simulink model "gesamtmodell"  (Simulink 7.9)
settings: Solver=ode45  StartTime=0.0  StopTime=6.5  RelTol=1e-3
values from neighbouring files (symbols this model uses):
  bias = [0;0;0]    [init.m]
  g = 9.81    [init.m]
  Kd = 4    [init.m]
  Ki = 0.01    [init.m]
  Kp = 5    [init.m]
  l_1 = 18    [init.m]
  l_2 = 46.18    [init.m]
  l_3 = 3.75    [init.m]
  m = 1.863    [init.m]
  omega_0 = 1.5    [init.m]
  xi = 1    [init.m]
libraries: simulink x4
settings Model: Creator=Matthias  LastModifiedBy=Matthias

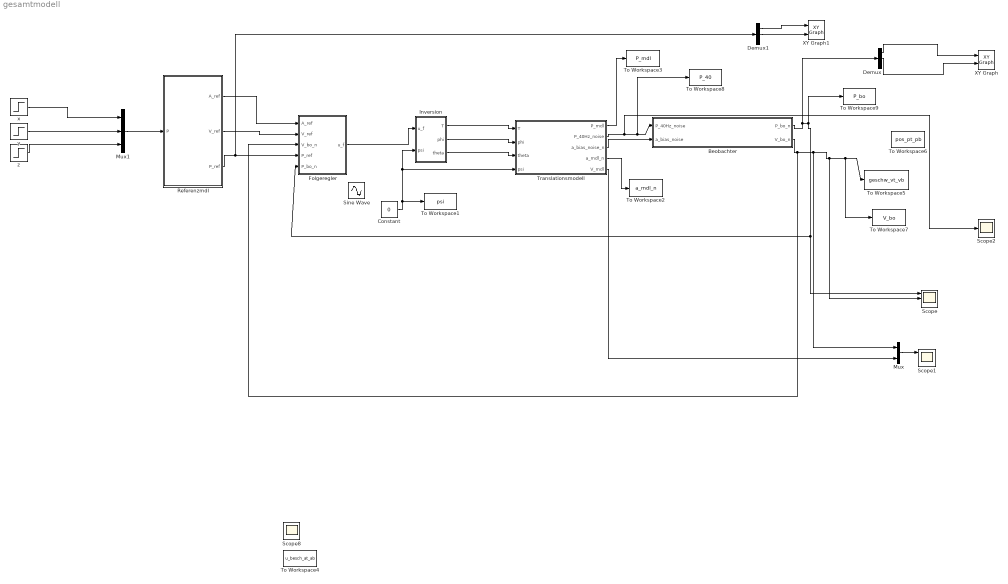
== system gesamtmodell ==
  Beobachter : Subsystem
  Constant : Constant  Value=0
  Demux : Demux  Outputs=3
  Demux1 : Demux  Outputs=3
  Folgeregler : Subsystem
  Inversion : Subsystem
  Mux : Mux  Inputs=2
  Mux1 : Mux  Inputs=3
  Referenzmdl : Subsystem
  Scope : Scope  NumInputPorts=3
      settings: TimeRange=7  YMin=-5~-5~-5  YMax=5~5~5
  Scope1 : Scope  NumInputPorts=3
      settings: YMin=-1.25~-5~-5  YMax=0.75~5~5
  Scope2 : Scope
      settings: SaveName=ScopeData6
  Scope8 : Scope
      settings: SaveName=ScopeData11
  Sine Wave : Sin  SampleTime=0
  To Workspace1 : ToWorkspace  VariableName=psi  SampleTime=-1  SaveFormat=Structure With Time
  To Workspace2 : ToWorkspace  VariableName=a_mdl_n  SampleTime=-1  SaveFormat=Structure With Time
  To Workspace3 : ToWorkspace  VariableName=P_mdl  SampleTime=-1  SaveFormat=Structure With Time
  To Workspace4 : ToWorkspace  VariableName=u_besch_at_ab  SampleTime=-1  SaveFormat=Structure With Time
  To Workspace5 : ToWorkspace  VariableName=geschw_vt_vb  SampleTime=-1  SaveFormat=Structure With Time
  To Workspace6 : ToWorkspace  VariableName=pos_pt_pb  SampleTime=-1  SaveFormat=Structure With Time
  To Workspace7 : ToWorkspace  VariableName=V_bo  SampleTime=-1  SaveFormat=Structure With Time
  To Workspace8 : ToWorkspace  VariableName=P_40  SampleTime=-1  SaveFormat=Structure With Time
  To Workspace9 : ToWorkspace  VariableName=P_bo  SampleTime=-1  SaveFormat=Structure With Time
  Translationsmodell : Subsystem
  XY Graph : simulink/Sinks/XY Graph  xmin=-2.5  xmax=0.5  ymin=-0.5  ymax=2.5  st=-1
  XY Graph1 : simulink/Sinks/XY Graph  xmin=-2.5  xmax=0.5  ymin=-0.5  ymax=2.5  st=-1
  x : Step  Time=0.5  After=-2  SampleTime=0
  y : Step  Time=0.5  SampleTime=0
  z : Step  After=0  SampleTime=0
  wires:
  Inversion/1(T) -> Translationsmodell/1(T)
  Inversion/2(phi) -> Translationsmodell/2(phi)
  Inversion/3(theta) -> Translationsmodell/3(theta)
  Translationsmodell/4(a_mdl_n) -> To Workspace2/1
  Translationsmodell/2(P_40Hz_noise) -> Scope2/1, Beobachter/1(P_40Hz_noise), To Workspace8/1
  Translationsmodell/3(a_bias_noise_n) -> Beobachter/2(a_bias_noise)
  Beobachter/2(V_bo_n) -> Scope/2, To Workspace5/1, To Workspace7/1, Mux/1, Folgeregler/3(V_bo_n)
  Mux1/1 -> Referenzmdl/1(P)
  Folgeregler/1(u_f) -> Inversion/1(u_f)
  Referenzmdl/1(A_ref) -> Folgeregler/1(A_ref)
  Referenzmdl/2(V_ref) -> Folgeregler/2(V_ref)
  Referenzmdl/3(P_ref) -> Folgeregler/4(P_ref), Demux1/1
  x/1 -> Mux1/1
  y/1 -> Mux1/2
  z/1 -> Mux1/3
  Translationsmodell/1(P_mdl) -> To Workspace3/1
  Translationsmodell/5(V_mdl) -> Mux/2
  Mux/1 -> Scope1/1
  Beobachter/1(P_bo_n) -> Demux/1, Scope/1, Folgeregler/5(P_bo_n), To Workspace9/1
  Demux/2 -> XY Graph/2
  Demux/1 -> XY Graph/1
  Demux1/1 -> XY Graph1/1
  Demux1/2 -> XY Graph1/2
  Constant/1 -> Inversion/2(psi), Translationsmodell/4(psi), To Workspace1/1

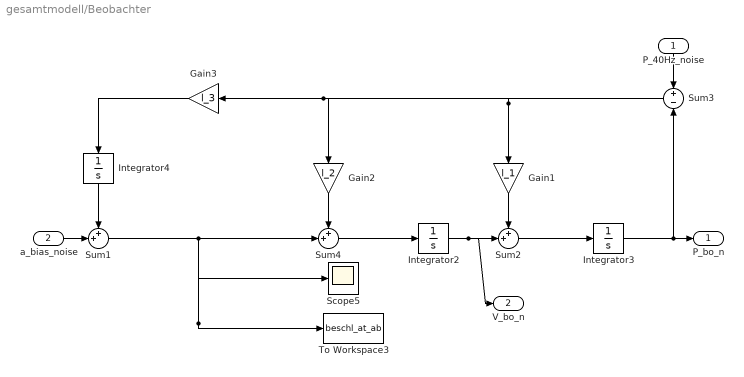
== system gesamtmodell/Beobachter ==
  P_40Hz_noise : Inport
  a_bias_noise : Inport  Port=2
  Gain1 : Gain  Gain=l_1
  Gain2 : Gain  Gain=l_2
  Gain3 : Gain  Gain=l_3
  Integrator2 : Integrator
  Integrator3 : Integrator
  Integrator4 : Integrator
  Scope5 : Scope
      settings: SaveName=ScopeData8
  Sum1 : Sum  Inputs=++|
  Sum2 : Sum  Inputs=++|
  Sum3 : Sum  Inputs=+|-
  Sum4 : Sum  Inputs=++|
  To Workspace3 : ToWorkspace  VariableName=beschl_at_ab  SampleTime=-1  SaveFormat=Structure With Time
  P_bo_n : Outport
  V_bo_n : Outport  Port=2
  wires:
  Gain3/1 -> Integrator4/1
  Sum1/1 -> Sum4/2, Scope5/1, To Workspace3/1
  Integrator4/1 -> Sum1/1
  Gain2/1 -> Sum4/1
  Sum4/1 -> Integrator2/1
  Sum3/1 -> Gain1/1, Gain3/1, Gain2/1
  Gain1/1 -> Sum2/1
  Integrator3/1 -> Sum3/2, P_bo_n/1
  Sum2/1 -> Integrator3/1
  Integrator2/1 -> Sum2/2, V_bo_n/1
  P_40Hz_noise/1 -> Sum3/1
  a_bias_noise/1 -> Sum1/2

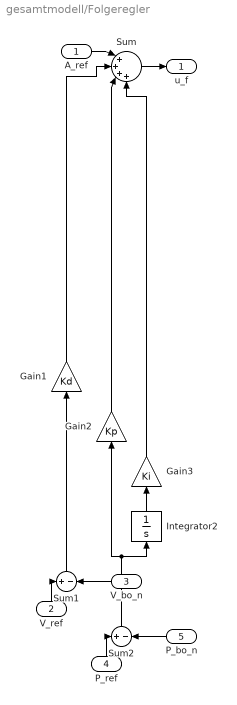
== system gesamtmodell/Folgeregler ==
  A_ref : Inport
  V_ref : Inport  Port=2
  V_bo_n : Inport  Port=3
  P_ref : Inport  Port=4
  P_bo_n : Inport  Port=5
  Gain1 : Gain  Gain=Kd
  Gain2 : Gain  Gain=Kp
  Gain3 : Gain  Gain=Ki
  Integrator2 : Integrator
  Sum : Sum  Inputs=|++++
  Sum1 : Sum  Inputs=+|-
  Sum2 : Sum  Inputs=+|-
  u_f : Outport
  wires:
  Sum1/1 -> Gain1/1
  Sum2/1 -> Gain2/1, Integrator2/1
  Integrator2/1 -> Gain3/1
  V_bo_n/1 -> Sum1/2
  P_bo_n/1 -> Sum2/2
  A_ref/1 -> Sum/1
  Sum/1 -> u_f/1
  V_ref/1 -> Sum1/1
  P_ref/1 -> Sum2/1
  Gain1/1 -> Sum/2
  Gain2/1 -> Sum/3
  Gain3/1 -> Sum/4

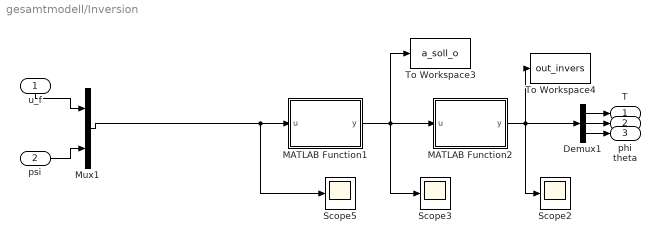
== system gesamtmodell/Inversion ==
  u_f : Inport
  psi : Inport  Port=2
  Demux1 : Demux  Outputs=3
  MATLAB Function1 : MATLAB Function  TreatAsAtomicUnit=on
  MATLAB Function2 : MATLAB Function  TreatAsAtomicUnit=on
  Mux1 : Mux  Inputs=2
  Scope2 : Scope
      settings: SaveName=ScopeData2
  Scope3 : Scope
      settings: SaveName=ScopeData3
  Scope5 : Scope
      settings: SaveName=ScopeData5
  To Workspace3 : ToWorkspace  VariableName=a_soll_o  SampleTime=-1  SaveFormat=Structure With Time
  To Workspace4 : ToWorkspace  VariableName=out_invers  SampleTime=-1  SaveFormat=Structure With Time
  T : Outport
  phi : Outport  Port=2
  theta : Outport  Port=3
  wires:
  Mux1/1 -> MATLAB Function1/1(u), Scope5/1
  MATLAB Function1/1(y) -> MATLAB Function2/1(u), Scope3/1, To Workspace3/1
  MATLAB Function2/1(y) -> Demux1/1, Scope2/1, To Workspace4/1
  u_f/1 -> Mux1/1
  psi/1 -> Mux1/2
  Demux1/1 -> T/1
  Demux1/2 -> phi/1
  Demux1/3 -> theta/1

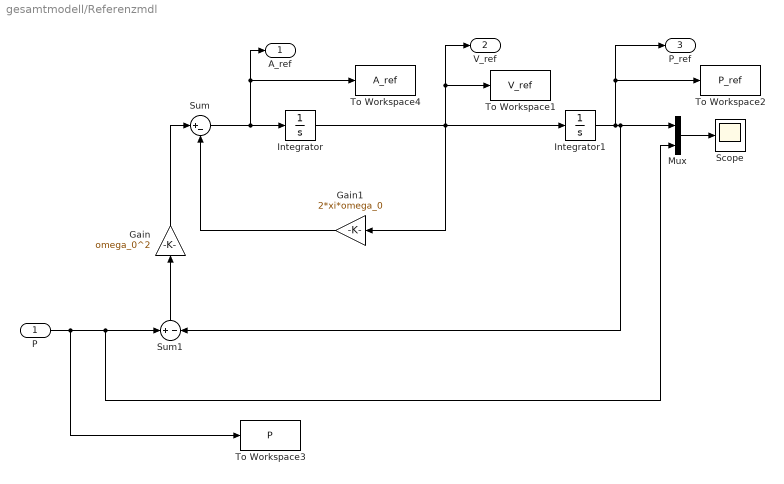
== system gesamtmodell/Referenzmdl ==
  P : Inport
  Gain : Gain  Gain=omega_0^2
  Gain1 : Gain  Gain=2*xi*omega_0
  Integrator : Integrator
  Integrator1 : Integrator
  Mux : Mux  Inputs=2
  Scope : Scope
  Sum : Sum  Inputs=|+-
  Sum1 : Sum  Inputs=+|-
  To Workspace1 : ToWorkspace  VariableName=V_ref  SampleTime=-1  SaveFormat=Structure With Time
  To Workspace2 : ToWorkspace  VariableName=P_ref  SampleTime=-1  SaveFormat=Structure With Time
  To Workspace3 : ToWorkspace  VariableName=P  SampleTime=-1  SaveFormat=Structure With Time
  To Workspace4 : ToWorkspace  VariableName=A_ref  SampleTime=-1  SaveFormat=Structure With Time
  A_ref : Outport
  V_ref : Outport  Port=2
  P_ref : Outport  Port=3
  wires:
  Sum1/1 -> Gain/1
  Gain/1 -> Sum/1
  Sum/1 -> Integrator/1, A_ref/1, To Workspace4/1
  Integrator/1 -> Integrator1/1, Gain1/1, V_ref/1, To Workspace1/1
  Gain1/1 -> Sum/2
  Integrator1/1 -> Sum1/2, Mux/1, P_ref/1, To Workspace2/1
  Mux/1 -> Scope/1
  P/1 -> Sum1/1, Mux/2, To Workspace3/1

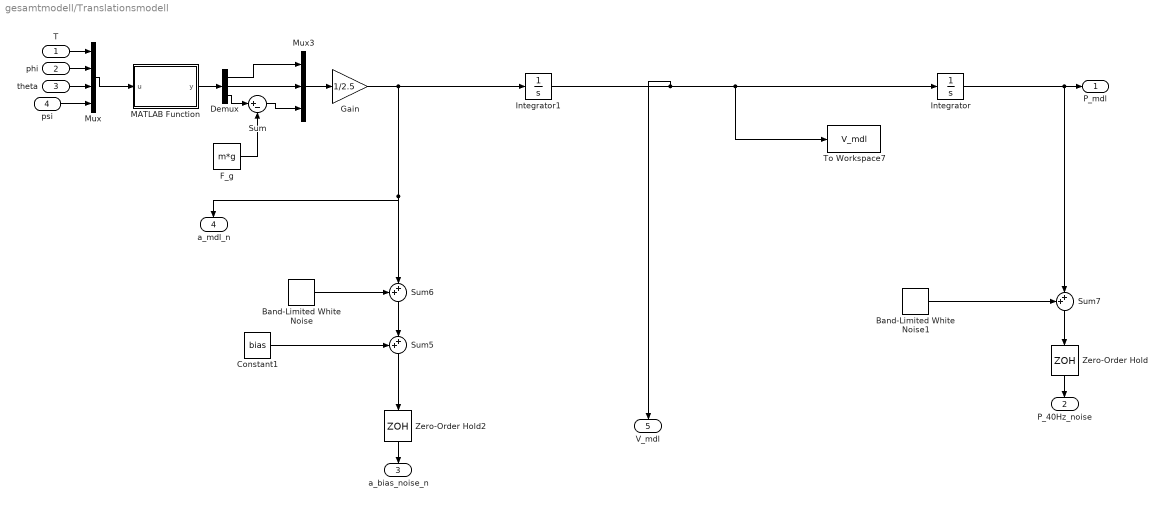
== system gesamtmodell/Translationsmodell ==
  T : Inport
  phi : Inport  Port=2
  theta : Inport  Port=3
  psi : Inport  Port=4
  Band-Limited White Noise : simulink/Sources/Band-Limited White Noise  Cov=[0.00001]  Ts=0.001  seed=[23341]
  Band-Limited White Noise1 : simulink/Sources/Band-Limited White Noise  Cov=[0.00005]  Ts=0.025  seed=[23341]
  Constant1 : Constant  Value=bias
  Demux : Demux  Outputs=3
  F_g : Constant  Value=m*g
  Gain : Gain  Gain=1/2.5
  Integrator : Integrator
  Integrator1 : Integrator
  MATLAB Function : MATLAB Function  TreatAsAtomicUnit=on
  Mux : Mux
  Mux3 : Mux  Inputs=3
  Sum : Sum  Inputs=|+-
  Sum5 : Sum  Inputs=++|
  Sum6 : Sum  Inputs=++|
  Sum7 : Sum  Inputs=++|
  To Workspace7 : ToWorkspace  VariableName=V_mdl  SampleTime=-1  SaveFormat=Structure With Time
  Zero-Order Hold : ZeroOrderHold  SampleTime=.025
  Zero-Order Hold2 : ZeroOrderHold  SampleTime=.001
  P_mdl : Outport
  P_40Hz_noise : Outport  Port=2
  a_bias_noise_n : Outport  Port=3
  a_mdl_n : Outport  Port=4
  V_mdl : Outport  Port=5
  wires:
  Integrator1/1 -> Integrator/1, To Workspace7/1, V_mdl/1
  Integrator/1 -> Sum7/2, P_mdl/1
  Gain/1 -> Integrator1/1, Sum6/2, a_mdl_n/1
  Mux/1 -> MATLAB Function/1(u)
  MATLAB Function/1(y) -> Demux/1
  Demux/3 -> Sum/1
  F_g/1 -> Sum/2
  Demux/1 -> Mux3/1
  Demux/2 -> Mux3/2
  Sum/1 -> Mux3/3
  Mux3/1 -> Gain/1
  Constant1/1 -> Sum5/1
  Sum5/1 -> Zero-Order Hold2/1
  Sum6/1 -> Sum5/2
  Band-Limited White Noise/1 -> Sum6/1
  Sum7/1 -> Zero-Order Hold/1
  Band-Limited White Noise1/1 -> Sum7/1
  psi/1 -> Mux/4
  T/1 -> Mux/1
  phi/1 -> Mux/2
  theta/1 -> Mux/3
  Zero-Order Hold/1 -> P_40Hz_noise/1
  Zero-Order Hold2/1 -> a_bias_noise_n/1

== matlab function Inversion/MATLAB Function1 ==
  data: u input double; y output double
function y = fcn(u)
a_nx = u(1);
a_ny = u(2);
a_nz = u(3);
psi  = u(4);

Mz = [cos(psi) sin(psi) 0; -sin(psi) cos(psi) 0; 0 0 1;];
y = Mz * [a_nx;a_ny;a_nz];

== matlab function Translationsmodell/MATLAB Function ==
  data: u input double; y output double
function y = fcn(u)
T       = u(1);
phi     = u(2);
theta   = u(3);
psi     = u(4);

Mt = [cos(theta) * cos(psi) sin(phi) * sin(theta) * cos(psi) - cos(phi) * sin(psi) cos(phi) * sin(theta) * cos(psi) + sin(phi) * sin(psi); cos(theta) * sin(psi) sin(phi) * sin(theta) * sin(psi) + cos(phi) * cos(psi) cos(phi) * sin(theta) * sin(psi) - sin(phi) * cos(psi); -sin(theta) sin(phi) * cos(theta) cos(phi) * cos(theta);];


y = Mt * [0; 0; T];

== matlab function Inversion/MATLAB Function2 ==
  data: u input double; y output double
function y = fcn(u)
a_ox = u(1);
a_oy = u(2);
a_oz = u(3);
m = 1.863;
g = 9.81;


T       = m*(sqrt(a_ox^2+a_oy^2+(a_oz+g)^2));
phi     = asin(-(a_oy*m)/T);

theta   = atan(a_ox/(a_oz+g));

y = [T;phi;theta];
